simulink model "HydrogenRefuelingStation_Param"  (R2023b)
settings: Solver=VariableStepAuto  StartTime=0.0  StopTime=finSimulation  RelTol=1e-3  AbsTol=1e-3
PreLoadFcn:
  | load hydrogen_properties.mat
  | load silicone_fluid_properties.mat
  | 
  | p_storage = 200; % [bar]
  | p_vehicle_init = 100; % [bar]
  | T_env = 25; % [degC]
  | T_fluid = -60; % [degC]
  | 
  | V_vehicle = 172; % [l]
  | 
  | tube_D = 0.04; % [m]
  | hose_D = 0.0064; % [m]
  | pipe_D = 0.1; % [m]
  | 
  | num_buffer = 2;
  | 
  | intercooler_num_tubes = 25;
  | intercooler_tube_D = 0.008; % [m]
  | intercooler_shell_D = 0.1; % [m]
  | intercooler_L = 2; % [m]
  | 
  | precooler_tube_W = 0.001; % [m]
  | precooler_num_tubes = 50*25;
  | precooler_L = 1; % [m]
values from neighbouring files (symbols this model uses):
  EngDemandTime = 3000    [launch.m]
  EngThrottle = 1    [launch.m]
  ext_bufferEng_D = 0.025    [System_Parameters.m]
  ext_Manifold_D = 0.007    [System_Parameters.m]
  ext_vehTank_D = 0.25    [System_Parameters.m]
  in_bufferEng_D = 0.0064    [System_Parameters.m]
  in_Eng_D = 0.0064    [System_Parameters.m]
  in_Man_D = 0.0064    [System_Parameters.m]
  inOut_vehTank_D = 0.0064    [System_Parameters.m]
  int_bufferEng_D = 0.024    [System_Parameters.m]
  int_Manifold_D = 0.0064    [System_Parameters.m]
  int_vehTank_D = 0.22    [System_Parameters.m]
  L_bufferEng = 1    [System_Parameters.m]
  L_Manifold = 1    [System_Parameters.m]
  L_vehTank = 2    [System_Parameters.m]
  MV_D = 0.0064    [System_Parameters.m]
  out_bufferEng_D = 0.0064/2    (= 0.0032)    [System_Parameters.m]
  out_Eng_D = 0.0064    [System_Parameters.m]
  out_Man_D = 0.0064    [System_Parameters.m]
  Pipe_ConnMan_D = 0.0064    [System_Parameters.m]
  Pipe_ManPR_D = 0.0064    [System_Parameters.m]
  Pipe_ManTank_D = 0.0064    [System_Parameters.m]
  Pipe_PRBuffer_D = 0.0064    [System_Parameters.m]
  redn_PR_D = 0.0064    [System_Parameters.m]
  redn_PR_setP = 160    [System_Parameters.m]
  relief_PR_D = 0.0064    [System_Parameters.m]
  relief_vehTank_D = 0.0064    [System_Parameters.m]
  silicone_fluid =     [silicone_fluid_properties.mat]
  statConn_D = 0.0064    [System_Parameters.m]
  stationTrigger_Time = 2400    [System_Parameters.m]
  SV_D = 0.0064    [System_Parameters.m]
  tank_Man_D = 0.0064    [System_Parameters.m]
  TempCont_vehTank_D = 0.0064    [System_Parameters.m]
  vehConn_D = 0.0064    [System_Parameters.m]
  WP_high = 700    [System_Parameters.m]
libraries: fl_lib x128, nesl_utility x60, SimscapeFluids_lib x41, slpidlib x4
(part 3 of 6)

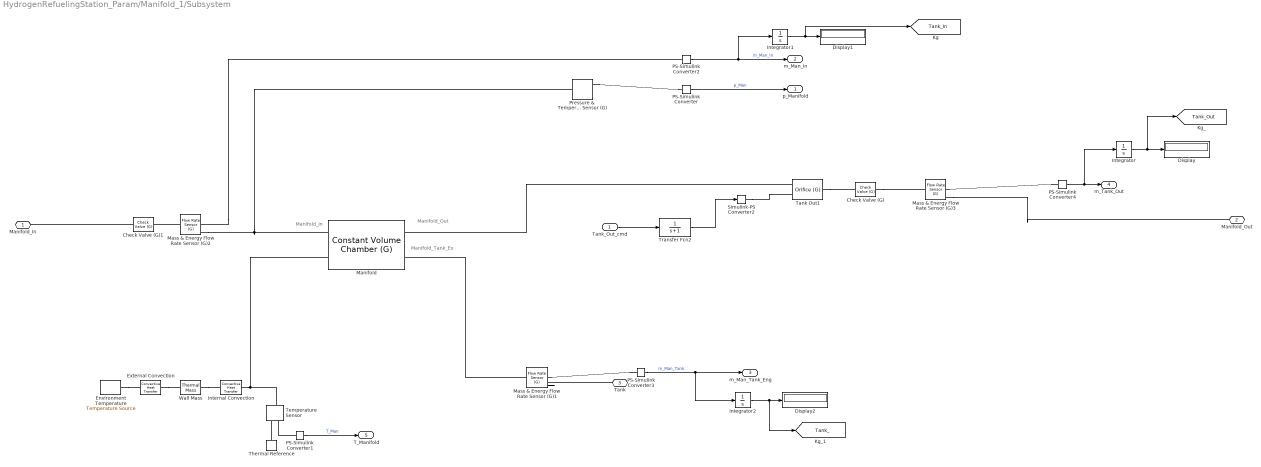
== system HydrogenRefuelingStation_Param/Manifold_1/Subsystem ==
  note: Manifold_In
  note: Manifold_Tank_Ex
  note: Manifold_Out
  Tank_Out_cmd : Inport
  Check Valve (G) : SimscapeFluids_lib/Gas/Valves & Orifices/Directional Control Valves/Check Valve (G)  opening_pressure_spec=fluids.gas.valves_orifices.enum.PressureControlSpec.PressureA  p_crack_differential=0.01 MPa  p_crack_gauge=0.1 bar  press_max_differential=70 MPa  press_max_gauge=WP_high + 50 bar  valve_parameterization=fluids.gas.valves_orifices.enum.OrificeParameterization.Cv  Cv_max=0.8  xT_Cv=0.7  Kv_max=3.6  xT_Kv=0.7  C_max=12 l/(bar*s)  B_crit_linear=0.3  m=0.5  T_ref_C=293.15 K  rho_ref_C=1.185 kg/m^3  orifice_area_max=1e-4 m^2  Cd=0.64  leakage_fraction=1e-6  smoothing_factor=0.01  B_lam=0.999  area=pi*out_Man_D^2/4 m^2
      settings: InternalSimscapePortConfiguration="{\"Bottom\":[],\"Left\":[{\"id\":\"A\",\"label\":\"A\",\"type\":\"foundation.gas.gas\"}],\"Right\":[{\"id\":\"B\",\"label\":\"B\",\"type\":\"foundation.gas.gas\"}],\"Top\":[]}"
  Check Valve (G)1 : SimscapeFluids_lib/Gas/Valves & Orifices/Directional Control Valves/Check Valve (G)  opening_pressure_spec=fluids.gas.valves_orifices.enum.PressureControlSpec.PressureA  p_crack_differential=0.01 MPa  p_crack_gauge=1 bar  press_max_differential=0.1 MPa  press_max_gauge=WP_high + 50 bar  valve_parameterization=fluids.gas.valves_orifices.enum.OrificeParameterization.Cv  Cv_max=4  xT_Cv=0.7  Kv_max=3.6  xT_Kv=0.7  C_max=12 l/(bar*s)  B_crit_linear=0.3  m=0.5  T_ref_C=293.15 K  rho_ref_C=1.185 kg/m^3  orifice_area_max=1e-4 m^2  Cd=0.64  leakage_fraction=1e-6  smoothing_factor=0.01  B_lam=0.999  area=pi*in_Man_D^2/4 m^2
      settings: InternalSimscapePortConfiguration="{\"Bottom\":[],\"Left\":[{\"id\":\"A\",\"label\":\"A\",\"type\":\"foundation.gas.gas\"}],\"Right\":[{\"id\":\"B\",\"label\":\"B\",\"type\":\"foundation.gas.gas\"}],\"Top\":[]}"
  Display : Display
  Display1 : Display
  Display2 : Display
  Environment Temperature : fl_lib/Thermal/Thermal Sources/Temperature Source  temperature=T_env degC
  External Convection : fl_lib/Thermal/Thermal Elements/Convective Heat Transfer  thermal_type=foundation.enum.constant_variable.constant  area=2*pi*(ext_Manifold_D/2)*L_Manifold m^2  heat_tr_coeff=h_ext_Manifold W/(K*m^2)  min_heat_tr_coeff=1e-3 W/(K*m^2)  T_specify=off  T_priority=None  T=0 K  T_nominal_specify=off  T_nominal_unit=K  T_nominal_value=1  Q_specify=off  Q_priority=None  Q=0 W  Q_nominal_specify=off  Q_nominal_unit=W  Q_nominal_value=1
  Integrator : Integrator
  Integrator1 : Integrator
  Integrator2 : Integrator
  Internal Convection : fl_lib/Thermal/Thermal Elements/Convective Heat Transfer  thermal_type=foundation.enum.constant_variable.constant  area=2*pi*(int_Manifold_D/2)*L_Manifold m^2  heat_tr_coeff=h_int_Manifold W/(K*m^2)  min_heat_tr_coeff=1e-3 W/(K*m^2)  T_specify=off  T_priority=None  T=0 K  T_nominal_specify=off  T_nominal_unit=K  T_nominal_value=1  Q_specify=off  Q_priority=None  Q=0 W  Q_nominal_specify=off  Q_nominal_unit=W  Q_nominal_value=1
  Manifold : fl_lib/Gas/Elements/Constant Volume Chamber (G)  volume=V_manifold l  num_ports=foundation.enum.num_ports.three  area_A=pi*in_Man_D^2/4 m^2  area_B=pi*out_Man_D^2/4 m^2  area_C=pi*tank_Man_D^2/4 m^2  area_D=0.01 m^2  p_I_specify=on  p_I_priority=High  p_I=p_vehTank_init bar  p_I_nominal_specify=off  p_I_nominal_unit=MPa  p_I_nominal_value=1  T_I_specify=on  T_I_priority=High  T_I=T_env degC  T_I_nominal_specify=off  T_I_nominal_unit=K  T_I_nominal_value=1  rho_I_specify=off  rho_I_priority=None  rho_I=1.2 kg/m^3  rho_I_nominal_specify=off  rho_I_nominal_unit=kg/m^3  rho_I_nominal_value=1
      settings: InternalSimscapePortConfiguration="{\"Bottom\":[],\"Left\":[{\"id\":\"A\",\"label\":\"A\",\"type\":\"foundation.gas.gas\"},{\"id\":\"H\",\"label\":\"H\",\"type\":\"foundation.thermal.thermal\"}],\"Right\":[{\"id\":\"B\",\"label\":\"B\",\"type\":\"foundation.gas.gas\"},{\"id\":\"C\",\"label\":\"C\",\"type\":\"foundation.gas.gas\"}],\"Top\":[]}"
  Mass & Energy Flow Rate Sensor (G)1 : fl_lib/Gas/Sensors/Flow Rate Sensor (G)  mass_flow_measure=true  volumetric_flow_measure=false  volumetric_flow_conditions=foundation.enum.volumetric_flow_conditions.actual  p_std=0.101325 MPa  T_std=20 degC  energy_flow_measure=true
      settings: InternalSimscapePortConfiguration="{\"Bottom\":[{\"id\":\"PHI\",\"label\":\"φ\",\"type\":\"output\"}],\"Left\":[{\"id\":\"A\",\"label\":\"A\",\"type\":\"foundation.gas.gas\"}],\"Right\":[{\"id\":\"B\",\"label\":\"B\",\"type\":\"foundation.gas.gas\"},{\"id\":\"M\",\"label\":\"M\",\"type\":\"output\"}],\"Top\":[]}"
  Mass & Energy Flow Rate Sensor (G)2 : fl_lib/Gas/Sensors/Flow Rate Sensor (G)  mass_flow_measure=true  volumetric_flow_measure=false  volumetric_flow_conditions=foundation.enum.volumetric_flow_conditions.actual  p_std=0.101325 MPa  T_std=20 degC  energy_flow_measure=true
      settings: InternalSimscapePortConfiguration="{\"Bottom\":[{\"id\":\"PHI\",\"label\":\"φ\",\"type\":\"output\"}],\"Left\":[{\"id\":\"A\",\"label\":\"A\",\"type\":\"foundation.gas.gas\"}],\"Right\":[{\"id\":\"B\",\"label\":\"B\",\"type\":\"foundation.gas.gas\"},{\"id\":\"M\",\"label\":\"M\",\"type\":\"output\"}],\"Top\":[]}"
  Mass & Energy Flow Rate Sensor (G)3 : fl_lib/Gas/Sensors/Flow Rate Sensor (G)  mass_flow_measure=true  volumetric_flow_measure=false  volumetric_flow_conditions=foundation.enum.volumetric_flow_conditions.actual  p_std=0.101325 MPa  T_std=20 degC  energy_flow_measure=true
      settings: InternalSimscapePortConfiguration="{\"Bottom\":[{\"id\":\"PHI\",\"label\":\"φ\",\"type\":\"output\"}],\"Left\":[{\"id\":\"A\",\"label\":\"A\",\"type\":\"foundation.gas.gas\"}],\"Right\":[{\"id\":\"B\",\"label\":\"B\",\"type\":\"foundation.gas.gas\"},{\"id\":\"M\",\"label\":\"M\",\"type\":\"output\"}],\"Top\":[]}"
  PS-Simulink Converter : nesl_utility/PS-Simulink Converter  PhysicalDomain=network_engine_domain  SubClassName=ps_output  LeftPortType=input  RightPortType=output  PseudoPeriodic=off  Frequencies=[]  VectorFormat=inherit  Unit=bar  AffineConversion=off
  PS-Simulink Converter1 : nesl_utility/PS-Simulink Converter  PhysicalDomain=network_engine_domain  SubClassName=ps_output  LeftPortType=input  RightPortType=output  PseudoPeriodic=off  Frequencies=[]  VectorFormat=inherit  Unit=degC  AffineConversion=on
  PS-Simulink Converter2 : nesl_utility/PS-Simulink Converter  PhysicalDomain=network_engine_domain  SubClassName=ps_output  LeftPortType=input  RightPortType=output  PseudoPeriodic=off  Frequencies=[]  VectorFormat=inherit  Unit=kg/s  AffineConversion=off
  PS-Simulink Converter3 : nesl_utility/PS-Simulink Converter  PhysicalDomain=network_engine_domain  SubClassName=ps_output  LeftPortType=input  RightPortType=output  PseudoPeriodic=off  Frequencies=[]  VectorFormat=inherit  Unit=kg/s  AffineConversion=off
  PS-Simulink Converter4 : nesl_utility/PS-Simulink Converter  PhysicalDomain=network_engine_domain  SubClassName=ps_output  LeftPortType=input  RightPortType=output  PseudoPeriodic=off  Frequencies=[]  VectorFormat=inherit  Unit=kg/s  AffineConversion=off
  Pressure & Temperature Sensor (G) : fl_lib/Gas/Sensors/Pressure & Temperature Sensor (G)  reference=foundation.enum.MeasurementReference.absolute  pressure=true  pressure_spec=foundation.enum.PressureMeasementSpec.Absolute  temperature=true
      settings: InternalSimscapePortConfiguration="{\"Bottom\":[{\"id\":\"T\",\"label\":\"T\",\"type\":\"output\"}],\"Left\":[{\"id\":\"A\",\"label\":\"A\",\"type\":\"foundation.gas.gas\"}],\"Right\":[{\"id\":\"Pa\",\"label\":\"Pa\",\"type\":\"output\"}],\"Top\":[]}"
  Simulink-PS Converter2 : nesl_utility/Simulink-PS Converter  PhysicalDomain=network_engine_domain  SubClassName=ps_input  LeftPortType=input  RightPortType=output  PseudoPeriodic=off  Frequencies=[]  NoiseDistribution=none  NoiseParameters=[]  Unit=1  AffineConversion=off  FilteringAndDerivatives=provide  SimscapeFilterOrder=1  InputFilterTimeConstant=0.001  UdotUserProvided=0
  Tank Out1 : SimscapeFluids_lib/Gas/Valves & Orifices/Orifice (G)  orifice_type=foundation.enum.constant_variable.variable  orifice_parameterization=fluids.gas.valves_orifices.enum.OrificeParameterization.Cv  opening_characteristic=fluids.gas.valves_orifices.enum.OpeningCharacteristics.Linear  Cv_constant=4  Cv_max=0.8  L_Cv_TLU=0 : 0.2 : 1  Cv_TLU=[1e-06, .8, 1.6, 2.4, 3.2, 4]  xT_Cv=0.7  Kv_constant=3.6  Kv_max=3.6  L_Kv_TLU=0 : 0.2 : 1  Kv_TLU=[1e-06, .72, 1.44, 2.16, 2.88, 3.6]  xT_Kv=0.7  C_constant=12 l/(bar*s)  B_crit_constant=0.3  C_max=12 l/(bar*s)  B_crit_linear=0.3  L_C_TLU=0 : 0.2 : 1  C_TLU=[1e-05, 2.4, 4.8, 7.2, 9.6, 12] l/(bar*s)  B_crit_TLU=0.3 * ones(1, 6)  m=0.5  T_ref_C=293.15 K  rho_ref_C=1.185 kg/m^3  orifice_area_constant=1e-4 m^2  orifice_area_max=1e-4 m^2  L_orifice_area_TLU=0 : 0.2 : 1  orifice_area_TLU=[1e-10, 2e-05, 4e-05, 6e-05, 8e-05, .0001] m^2  Cd=0.64  leakage_fraction=1e-6  smoothing_factor=0  B_lam=0.999  area=pi*out_Man_D^2/4 m^2
      settings: InternalSimscapePortConfiguration="{\"Bottom\":[],\"Left\":[{\"id\":\"A\",\"label\":\"A\",\"type\":\"foundation.gas.gas\"},{\"id\":\"L\",\"label\":\"L\",\"type\":\"input\"}],\"Right\":[{\"id\":\"B\",\"label\":\"B\",\"type\":\"foundation.gas.gas\"}],\"Top\":[]}"
  Temperature Sensor : fl_lib/Thermal/Thermal Sensors/Temperature Sensor  temperature_measure=foundation.enum.MeasurementReference.difference
  Thermal Reference : fl_lib/Thermal/Thermal Elements/Thermal Reference
  Transfer Fcn2 : TransferFcn  Denominator=[1 1]
  Wall Mass : fl_lib/Thermal/Thermal Elements/Thermal Mass  mass_type=foundation.enum.constant_variable.constant  mass=M_Manifold kg  sp_heat=c_Manifold J/(K*kg)  mass_min=1e-6 kg  num_ports=foundation.enum.numPorts2.two  m_specify=off  m_priority=High  m=1 kg  m_nominal_specify=off  m_nominal_unit=kg  m_nominal_value=1  T_specify=on  T_priority=High  T=T_env degC  T_nominal_specify=off  T_nominal_unit=K  T_nominal_value=1  Q_specify=off  Q_priority=None  Q=0 W  Q_nominal_specify=off  Q_nominal_unit=W  Q_nominal_value=1
      settings: InternalSimscapePortConfiguration="{\"Bottom\":[],\"Left\":[{\"id\":\"M\",\"label\":\"\",\"type\":\"foundation.thermal.thermal\"}],\"Right\":[{\"id\":\"N\",\"label\":\"\",\"type\":\"foundation.thermal.thermal\"}],\"Top\":[]}"
  Manifold_In : PMIOPort  Side=Left
  Manifold_Out : PMIOPort  Port=2  Side=Right
  Tank : PMIOPort  Port=3  Side=Right
  p_Manifold : Outport
  m_Man_In : Outport  Port=2
  m_Man_Tank_Eng : Outport  Port=3
  m_Tank_Out : Outport  Port=4
  T_Manifold : Outport  Port=5
  tag scope: Tank_=global, Tank_In=global, Tank_Out=global
  wires:
  PS-Simulink Converter4/1 -> Integrator/1, m_Tank_Out/1
  PS-Simulink Converter2/1 -> Integrator1/1, m_Man_In/1  "m_Man_In"
  Integrator1/1 -> [Tank_In], Display1/1
  Integrator/1 -> [Tank_Out], Display/1
  Transfer Fcn2/1 -> Simulink-PS Converter2/1
  PS-Simulink Converter3/1 -> Integrator2/1, m_Man_Tank_Eng/1  "m_Man_Tank"
  PS-Simulink Converter/1 -> p_Manifold/1  "p_Man"
  PS-Simulink Converter1/1 -> T_Manifold/1  "T_Man"
  Integrator2/1 -> [Tank_], Display2/1
  Tank_Out_cmd/1 -> Transfer Fcn2/1
  connections:
  Pressure & Temperature Sensor (G)/RConn1 -- PS-Simulink Converter/LConn1
  Check Valve (G)/RConn1 -- Mass & Energy Flow Rate Sensor (G)3/LConn1
  PS-Simulink Converter3/LConn1 -- Mass & Energy Flow Rate Sensor (G)1/RConn2
  PS-Simulink Converter2/LConn1 -- Mass & Energy Flow Rate Sensor (G)2/RConn2
  Mass & Energy Flow Rate Sensor (G)3/RConn1 -- Manifold_Out/RConn1
  External Convection/LConn1 -- Wall Mass/RConn1
  Mass & Energy Flow Rate Sensor (G)1/RConn1 -- Tank/RConn1
  Thermal Reference/LConn1 -- Temperature Sensor/RConn1
  PS-Simulink Converter4/LConn1 -- Mass & Energy Flow Rate Sensor (G)3/RConn2
  Tank Out1/RConn1 -- Check Valve (G)/LConn1
  Mass & Energy Flow Rate Sensor (G)2/LConn1 -- Check Valve (G)1/RConn1
  PS-Simulink Converter1/LConn1 -- Temperature Sensor/RConn2
  Internal Convection/LConn1 -- Temperature Sensor/LConn1 -- Manifold/LConn2
  Simulink-PS Converter2/RConn1 -- Tank Out1/LConn2
  Check Valve (G)1/LConn1 -- Manifold_In/RConn1
  Mass & Energy Flow Rate Sensor (G)2/RConn1 -- Manifold/LConn1 -- Pressure & Temperature Sensor (G)/LConn1
  Wall Mass/LConn1 -- Internal Convection/RConn1
  Environment Temperature/LConn1 -- External Convection/RConn1
  Mass & Energy Flow Rate Sensor (G)1/LConn1 -- Manifold/RConn2
  Tank Out1/LConn1 -- Manifold/RConn1

== system HydrogenRefuelingStation_Param/STATION/Cascade Buffer ==
  S_buffer : Inport
  Demux : Demux  Outputs=2
  High-Pressure : Subsystem  Tag=PublishSubsystem
      settings: PortSchema="{\"entries\":[{\"content\":{\"sides\":[{\"content\":{\"connectorIds\":[\"LConn1\"]},\"type\":\"ConnectorPlacement.EquallySpacedRectSide\",\"uuid\":\"b00ba4dd-6dda-4fc1-8418-16d977b72658\"},{\"content\":{\"connectorIds\":[\"RConn1\"],\"side\":\"RIGHT\"},\"type\":\"ConnectorPlacement.EquallySpacedRectSide\",\"uuid\":\"8ce3b878-20da-4ae3-b32b-b25a417e40c7\"},{\"content\":{\"connectorIds\":[\"Out1\",\"Out2\"],\"side\":\"TOP\"},\"type\":\"ConnectorPlacement.EquallySpacedRectSide\",\"uuid\":\"178fea87-568c-460e-ad58-627cda0af208\"},{\"content\":{\"connectorIds\":[],\"side\":\"BOTTOM\"},\"type\":\"ConnectorPlacement.EquallySpacedRectSide\",\"uuid\":\"da377dea-32af-4e40-bf21-9605c244d1e1\"}]},\"type\":\"ConnectorPlacement.EquallySpacedConnector\",\"uuid\":\"9a70e3bb-46a6-4db7-b9e8-afd83bfe5c73\"}],\"packageUris\":[\"http://schema.mathworks.com/mf0/Connector/R2020b\"],\"version\":\"1.0\"}"
  Low-Pressure : Subsystem
      settings: PortSchema="{\"entries\":[{\"content\":{\"sides\":[{\"content\":{\"connectorIds\":[\"LConn1\"]},\"type\":\"ConnectorPlacement.EquallySpacedRectSide\",\"uuid\":\"b00ba4dd-6dda-4fc1-8418-16d977b72658\"},{\"content\":{\"connectorIds\":[\"RConn1\"],\"side\":\"RIGHT\"},\"type\":\"ConnectorPlacement.EquallySpacedRectSide\",\"uuid\":\"8ce3b878-20da-4ae3-b32b-b25a417e40c7\"},{\"content\":{\"connectorIds\":[\"Out1\",\"Out2\"],\"side\":\"TOP\"},\"type\":\"ConnectorPlacement.EquallySpacedRectSide\",\"uuid\":\"178fea87-568c-460e-ad58-627cda0af208\"},{\"content\":{\"connectorIds\":[],\"side\":\"BOTTOM\"},\"type\":\"ConnectorPlacement.EquallySpacedRectSide\",\"uuid\":\"da377dea-32af-4e40-bf21-9605c244d1e1\"}]},\"type\":\"ConnectorPlacement.EquallySpacedConnector\",\"uuid\":\"9a70e3bb-46a6-4db7-b9e8-afd83bfe5c73\"}],\"packageUris\":[\"http://schema.mathworks.com/mf0/Connector/R2020b\"],\"version\":\"1.0\"}"
  Medium-Pressure : Subsystem
      settings: PortSchema="{\"entries\":[{\"content\":{\"sides\":[{\"content\":{\"connectorIds\":[\"LConn1\"]},\"type\":\"ConnectorPlacement.EquallySpacedRectSide\",\"uuid\":\"b00ba4dd-6dda-4fc1-8418-16d977b72658\"},{\"content\":{\"connectorIds\":[\"RConn1\"],\"side\":\"RIGHT\"},\"type\":\"ConnectorPlacement.EquallySpacedRectSide\",\"uuid\":\"8ce3b878-20da-4ae3-b32b-b25a417e40c7\"},{\"content\":{\"connectorIds\":[\"Out1\",\"Out2\"],\"side\":\"TOP\"},\"type\":\"ConnectorPlacement.EquallySpacedRectSide\",\"uuid\":\"178fea87-568c-460e-ad58-627cda0af208\"},{\"content\":{\"connectorIds\":[],\"side\":\"BOTTOM\"},\"type\":\"ConnectorPlacement.EquallySpacedRectSide\",\"uuid\":\"da377dea-32af-4e40-bf21-9605c244d1e1\"}]},\"type\":\"ConnectorPlacement.EquallySpacedConnector\",\"uuid\":\"9a70e3bb-46a6-4db7-b9e8-afd83bfe5c73\"}],\"packageUris\":[\"http://schema.mathworks.com/mf0/Connector/R2020b\"],\"version\":\"1.0\"}"
  Priority Valves In : Subsystem  Tag=PublishSubsystem
      settings: PortSchema="{\"entries\":[{\"content\":{\"sides\":[{\"content\":{\"connectorIds\":[\"LConn1\"]},\"type\":\"ConnectorPlacement.EquallySpacedRectSide\",\"uuid\":\"92348d24-87ef-48f7-b123-8d15e251ec5f\"},{\"content\":{\"connectorIds\":[\"RConn1\",\"RConn2\",\"RConn3\"],\"side\":\"RIGHT\"},\"type\":\"ConnectorPlacement.EquallySpacedRectSide\",\"uuid\":\"7c2c6e50-e97f-44c7-b52a-122ec7f82cb6\"},{\"content\":{\"connectorIds\":[\"In1\"],\"side\":\"TOP\"},\"type\":\"ConnectorPlacement.EquallySpacedRectSide\",\"uuid\":\"1dfda1f6-cfd2-4a29-b1d9-94627ecd7d6f\"}]},\"type\":\"ConnectorPlacement.EquallySpacedConnector\",\"uuid\":\"be7ce4ae-fd1d-4d31-a88b-a7c79f76950d\"}],\"packageUris\":[\"http://schema.mathworks.com/mf0/Connector/R2020b\"],\"version\":\"1.0\"}"
  Priority Valves Out : Subsystem
      settings: PortSchema="{\"entries\":[{\"content\":{\"sides\":[{\"content\":{\"connectorIds\":[\"LConn1\",\"LConn2\",\"LConn3\"]},\"type\":\"ConnectorPlacement.EquallySpacedRectSide\",\"uuid\":\"a55192f6-0bc3-43fb-9a62-e1a553f241a1\"},{\"content\":{\"connectorIds\":[\"RConn1\"],\"side\":\"RIGHT\"},\"type\":\"ConnectorPlacement.EquallySpacedRectSide\",\"uuid\":\"27038c48-7032-4a7e-b59b-b8c9e70a1ab2\"},{\"content\":{\"connectorIds\":[\"In1\"],\"side\":\"TOP\"},\"type\":\"ConnectorPlacement.EquallySpacedRectSide\",\"uuid\":\"7d646389-392e-44bb-96ea-475018d7fd6f\"}]},\"type\":\"ConnectorPlacement.EquallySpacedConnector\",\"uuid\":\"4d005342-a59b-47e4-b412-051eb9295e9d\"}],\"packageUris\":[\"http://schema.mathworks.com/mf0/Connector/R2020b\"],\"version\":\"1.0\"}"
  Scope : Scope
  Scope1 : Scope
  Vector Concatenate : Concatenate  NumInputs=3
  Vector Concatenate1 : Concatenate  NumInputs=3
  A : PMIOPort  Side=Left
  B : PMIOPort  Port=2  Side=Right
  p_buffer : Outport
  T_buffer : Outport  Port=2
  wires:
  Vector Concatenate/1 -> Scope/1, p_buffer/1
  High-Pressure/1(p) -> Vector Concatenate/1
  Medium-Pressure/1(p) -> Vector Concatenate/2
  Low-Pressure/1(p) -> Vector Concatenate/3
  S_buffer/1 -> Scope1/1, Demux/1
  Demux/1 -> Priority Valves In/1(S_buffer_in)
  Demux/2 -> Priority Valves Out/1(S_buffer_out)
  High-Pressure/2(T) -> Vector Concatenate1/1
  Medium-Pressure/2(T) -> Vector Concatenate1/2
  Low-Pressure/2(T) -> Vector Concatenate1/3
  Vector Concatenate1/1 -> T_buffer/1
  connections:
  Priority Valves In/LConn1 -- A/RConn1
  B/RConn1 -- Priority Valves Out/RConn1
  High-Pressure/LConn1 -- Priority Valves In/RConn1
  Priority Valves In/RConn2 -- Medium-Pressure/LConn1
  Priority Valves In/RConn3 -- Low-Pressure/LConn1
  Priority Valves Out/LConn1 -- High-Pressure/RConn1
  Priority Valves Out/LConn2 -- Medium-Pressure/RConn1
  Priority Valves Out/LConn3 -- Low-Pressure/RConn1

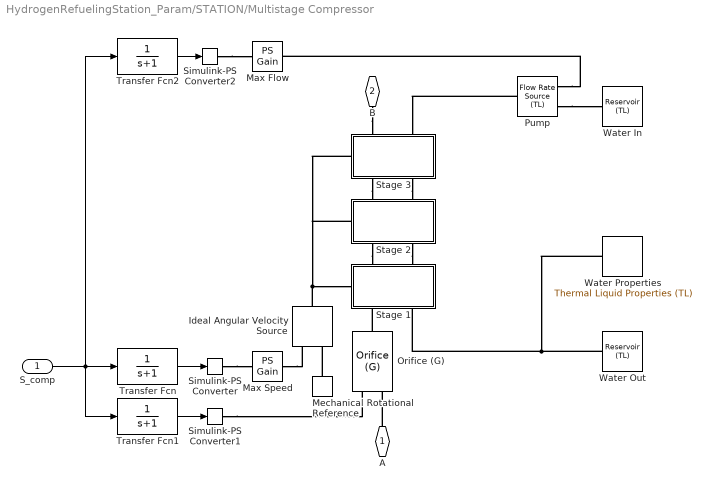
== system HydrogenRefuelingStation_Param/STATION/Multistage Compressor ==
  S_comp : Inport
  Ideal Angular Velocity Source : fl_lib/Mechanical/Mechanical Sources/Ideal Angular Velocity Source
  Max Flow : fl_lib/Physical Signals/Functions/PS Gain  gain=1.5 kg/s
  Max Speed : fl_lib/Physical Signals/Functions/PS Gain  gain=450 rpm
  Mechanical Rotational Reference : fl_lib/Mechanical/Rotational Elements/Mechanical Rotational Reference
  Orifice (G) : SimscapeFluids_lib/Gas/Valves & Orifices/Orifice (G)  orifice_type=foundation.enum.constant_variable.variable  orifice_parameterization=fluids.gas.valves_orifices.enum.OrificeParameterization.Cv  opening_characteristic=fluids.gas.valves_orifices.enum.OpeningCharacteristics.Linear  Cv_constant=4  Cv_max=0.8  L_Cv_TLU=0 : 0.2 : 1  Cv_TLU=[1e-06, .8, 1.6, 2.4, 3.2, 4]  xT_Cv=0.7  Kv_constant=3.6  Kv_max=3.6  L_Kv_TLU=0 : 0.2 : 1  Kv_TLU=[1e-06, .72, 1.44, 2.16, 2.88, 3.6]  xT_Kv=0.7  C_constant=12 l/(bar*s)  B_crit_constant=0.3  C_max=12 l/(bar*s)  B_crit_linear=0.3  L_C_TLU=0 : 0.2 : 1  C_TLU=[1e-05, 2.4, 4.8, 7.2, 9.6, 12] l/(bar*s)  B_crit_TLU=0.3 * ones(1, 6)  m=0.5  T_ref_C=293.15 K  rho_ref_C=1.185 kg/m^3  orifice_area_constant=1e-4 m^2  orifice_area_max=1e-4 m^2  L_orifice_area_TLU=0 : 0.2 : 1  orifice_area_TLU=[1e-10, 2e-05, 4e-05, 6e-05, 8e-05, .0001] m^2  Cd=0.64  leakage_fraction=1e-6  smoothing_factor=0  B_lam=0.999  area=pi*tube_D^2/4 m^2
      settings: InternalSimscapePortConfiguration="{\"Bottom\":[],\"Left\":[{\"id\":\"A\",\"label\":\"A\",\"type\":\"foundation.gas.gas\"},{\"id\":\"L\",\"label\":\"L\",\"type\":\"input\"}],\"Right\":[{\"id\":\"B\",\"label\":\"B\",\"type\":\"foundation.gas.gas\"}],\"Top\":[]}"
  Pump : fl_lib/Thermal Liquid/Sources/Flow Rate Source (TL)  source_type=foundation.enum.constant_controlled.controlled  flow_type=foundation.enum.mass_volumetric_flow.mass  mass_flow=0 kg/s  volumetric_flow=0 m^3/s  power_spec=foundation.enum.power_spec.isentropic  area=pi*pipe_D^2/4 m^2
  Simulink-PS Converter : nesl_utility/Simulink-PS Converter  PhysicalDomain=network_engine_domain  SubClassName=ps_input  LeftPortType=input  RightPortType=output  PseudoPeriodic=off  Frequencies=[]  NoiseDistribution=none  NoiseParameters=[]  Unit=1  AffineConversion=off  FilteringAndDerivatives=provide  SimscapeFilterOrder=1  InputFilterTimeConstant=0.001  UdotUserProvided=0
  Simulink-PS Converter1 : nesl_utility/Simulink-PS Converter  PhysicalDomain=network_engine_domain  SubClassName=ps_input  LeftPortType=input  RightPortType=output  PseudoPeriodic=off  Frequencies=[]  NoiseDistribution=none  NoiseParameters=[]  Unit=1  AffineConversion=off  FilteringAndDerivatives=provide  SimscapeFilterOrder=1  InputFilterTimeConstant=0.001  UdotUserProvided=0
  Simulink-PS Converter2 : nesl_utility/Simulink-PS Converter  PhysicalDomain=network_engine_domain  SubClassName=ps_input  LeftPortType=input  RightPortType=output  PseudoPeriodic=off  Frequencies=[]  NoiseDistribution=none  NoiseParameters=[]  Unit=1  AffineConversion=off  FilteringAndDerivatives=provide  SimscapeFilterOrder=1  InputFilterTimeConstant=0.001  UdotUserProvided=0
  Stage 1 : Subsystem  Tag=PublishSubsystem
      settings: PortSchema="{\"entries\":[{\"content\":{\"sides\":[{\"content\":{\"connectorIds\":[\"LConn1\"]},\"type\":\"ConnectorPlacement.EquallySpacedRectSide\",\"uuid\":\"cf2673b8-66bc-435b-b0d9-4d0b61a65baf\"},{\"content\":{\"connectorIds\":[],\"side\":\"RIGHT\"},\"type\":\"ConnectorPlacement.EquallySpacedRectSide\",\"uuid\":\"24b6c88b-0f30-49f8-a905-b89238d85e17\"},{\"content\":{\"connectorIds\":[\"LConn2\",\"LConn3\"],\"side\":\"TOP\"},\"type\":\"ConnectorPlacement.EquallySpacedRectSide\",\"uuid\":\"59149ba3-e6b1-4253-8751-c092b4d11562\"},{\"content\":{\"connectorIds\":[\"RConn1\",\"RConn2\"],\"side\":\"BOTTOM\"},\"type\":\"ConnectorPlacement.EquallySpacedRectSide\",\"uuid\":\"e5b3eee3-392f-4051-b3ca-9f847306bb8c\"}]},\"type\":\"ConnectorPlacement.EquallySpacedConnector\",\"uuid\":\"7d82cf02-c433-429f-849a-f8516d087c0d\"}],\"packageUris\":[\"http://schema.mathworks.com/mf0/Connector/R2020b\"],\"version\":\"1.0\"}"
  Stage 2 : Subsystem
      settings: PortSchema="{\"entries\":[{\"content\":{\"sides\":[{\"content\":{\"connectorIds\":[\"LConn1\"]},\"type\":\"ConnectorPlacement.EquallySpacedRectSide\",\"uuid\":\"cf2673b8-66bc-435b-b0d9-4d0b61a65baf\"},{\"content\":{\"connectorIds\":[],\"side\":\"RIGHT\"},\"type\":\"ConnectorPlacement.EquallySpacedRectSide\",\"uuid\":\"24b6c88b-0f30-49f8-a905-b89238d85e17\"},{\"content\":{\"connectorIds\":[\"LConn2\",\"LConn3\"],\"side\":\"TOP\"},\"type\":\"ConnectorPlacement.EquallySpacedRectSide\",\"uuid\":\"59149ba3-e6b1-4253-8751-c092b4d11562\"},{\"content\":{\"connectorIds\":[\"RConn1\",\"RConn2\"],\"side\":\"BOTTOM\"},\"type\":\"ConnectorPlacement.EquallySpacedRectSide\",\"uuid\":\"e5b3eee3-392f-4051-b3ca-9f847306bb8c\"}]},\"type\":\"ConnectorPlacement.EquallySpacedConnector\",\"uuid\":\"7d82cf02-c433-429f-849a-f8516d087c0d\"}],\"packageUris\":[\"http://schema.mathworks.com/mf0/Connector/R2020b\"],\"version\":\"1.0\"}"
  Stage 3 : Subsystem
      settings: PortSchema="{\"entries\":[{\"content\":{\"sides\":[{\"content\":{\"connectorIds\":[\"LConn1\"]},\"type\":\"ConnectorPlacement.EquallySpacedRectSide\",\"uuid\":\"cf2673b8-66bc-435b-b0d9-4d0b61a65baf\"},{\"content\":{\"connectorIds\":[],\"side\":\"RIGHT\"},\"type\":\"ConnectorPlacement.EquallySpacedRectSide\",\"uuid\":\"24b6c88b-0f30-49f8-a905-b89238d85e17\"},{\"content\":{\"connectorIds\":[\"LConn2\",\"LConn3\"],\"side\":\"TOP\"},\"type\":\"ConnectorPlacement.EquallySpacedRectSide\",\"uuid\":\"59149ba3-e6b1-4253-8751-c092b4d11562\"},{\"content\":{\"connectorIds\":[\"RConn1\",\"RConn2\"],\"side\":\"BOTTOM\"},\"type\":\"ConnectorPlacement.EquallySpacedRectSide\",\"uuid\":\"e5b3eee3-392f-4051-b3ca-9f847306bb8c\"}]},\"type\":\"ConnectorPlacement.EquallySpacedConnector\",\"uuid\":\"7d82cf02-c433-429f-849a-f8516d087c0d\"}],\"packageUris\":[\"http://schema.mathworks.com/mf0/Connector/R2020b\"],\"version\":\"1.0\"}"
  Transfer Fcn : TransferFcn  Denominator=[1 1]
  Transfer Fcn1 : TransferFcn  Denominator=[1 1]
  Transfer Fcn2 : TransferFcn  Denominator=[1 1]
  Water Properties : SimscapeFluids_lib/Thermal Liquid/Utilities/Thermal Liquid Properties (TL)  fluid_list=fluids.thermal_liquid.utilities.enum.thermal_liquid_fluid_list.water  concentration_param_EG=fluids.thermal_liquid.utilities.enum.thermal_liquid_concentration.volume_fraction  concentration_param_PG=fluids.thermal_liquid.utilities.enum.thermal_liquid_concentration.volume_fraction  c_mass_SW=3.5e-3  c_mass_EG=0.1  c_mass_PG=0.1  c_mass_GL=0.1  c_vol_EG=0.1  c_vol_PG=0.1  beta_const_EG=2.1791 GPa  beta_const_PG=2.1791 GPa  beta_const_GL=2.1791 GPa  p_min_EG=0.01 MPa  p_min_PG=0.01 MPa  p_min_GL=0.01 MPa  p_max_EG=50 MPa  p_max_PG=50 MPa  p_max_GL=50 MPa  p_atm=0.101325 MPa  properties_range_check=simscape.enum.assert.action.error
  Water In : fl_lib/Thermal Liquid/Elements/Reservoir (TL)  pressure_spec=foundation.enum.pressure_spec.atmospheric  reservoir_pressure=0.101325 MPa  reservoir_temperature=T_env degC  area=pi*pipe_D^2/4 m^2
  Water Out : fl_lib/Thermal Liquid/Elements/Reservoir (TL)  pressure_spec=foundation.enum.pressure_spec.atmospheric  reservoir_pressure=0.101325 MPa  reservoir_temperature=T_env degC  area=pi*pipe_D^2/4 m^2
  A : PMIOPort  Side=Left
  B : PMIOPort  Port=2  Side=Right
  wires:
  Transfer Fcn/1 -> Simulink-PS Converter/1
  Transfer Fcn1/1 -> Simulink-PS Converter1/1
  S_comp/1 -> Transfer Fcn2/1, Transfer Fcn1/1, Transfer Fcn/1
  Transfer Fcn2/1 -> Simulink-PS Converter2/1
  connections:
  Max Speed/RConn1 -- Ideal Angular Velocity Source/RConn1
  Pump/RConn1 -- Stage 3/LConn3
  Water Out/LConn1 -- Water Properties/RConn1 -- Stage 1/RConn2
  Stage 3/RConn1 -- Stage 2/LConn2
  Stage 3/RConn2 -- Stage 2/LConn3
  Stage 2/RConn1 -- Stage 1/LConn2
  Stage 2/RConn2 -- Stage 1/LConn3
  Mechanical Rotational Reference/LConn1 -- Ideal Angular Velocity Source/RConn2
  Simulink-PS Converter/RConn1 -- Max Speed/LConn1
  Ideal Angular Velocity Source/LConn1 -- Stage 3/LConn1 -- Stage 2/LConn1 -- Stage 1/LConn1
  B/RConn1 -- Stage 3/LConn2
  Orifice (G)/RConn1 -- Stage 1/RConn1
  A/RConn1 -- Orifice (G)/LConn1
  Simulink-PS Converter1/RConn1 -- Orifice (G)/LConn2
  Pump/LConn1 -- Water In/LConn1
  Simulink-PS Converter2/RConn1 -- Max Flow/LConn1
  Pump/LConn2 -- Max Flow/RConn1
